simulink model "closed_loop"  (R2019a)
settings: Solver=VariableStepAuto  StartTime=0.0  StopTime=10.0  RelTol=1e-3
values from neighbouring files (symbols this model uses):
  Kp_id = 10    [nomalization.m]
  r = 60    [nomalization.m]
  r_cyc = 4000*ts    (= 200)    [nomalization.m]
libraries: arduinolib x4
settings Model: Creator=xde12  LastModifiedBy=xde12

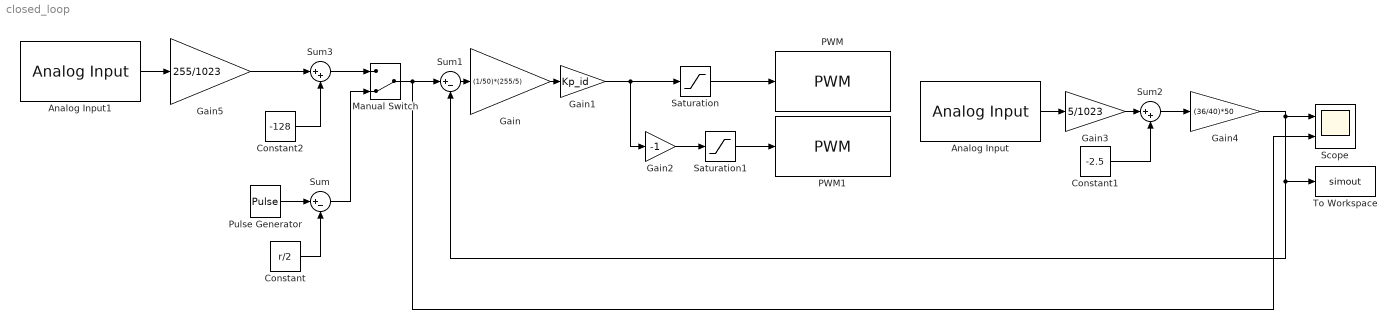
== system closed_loop ==
  Analog Input : arduinolib/Analog Input  pinNumber=0  ReadResultsOnly=off  ConversionTriggerSource=Software  ExternalTriggerType=uint32(0)  OutputDataType=uint16  EnableConversionCompleteNotify=off  EnableOuputStatus=off  SampleTime=0.01  blockPlatform=arduino
  Analog Input1 : arduinolib/Analog Input  pinNumber=0  ReadResultsOnly=off  ConversionTriggerSource=Software  ExternalTriggerType=uint32(0)  OutputDataType=uint16  EnableConversionCompleteNotify=off  EnableOuputStatus=off  SampleTime=0.01  blockPlatform=arduino
  Constant : Constant  Value=r/2  SampleTime=0.01
  Constant1 : Constant  Value=-2.5
  Constant2 : Constant  Value=-128  SampleTime=0.01
  Gain : Gain  Gain=(1/50)*(255/5)
  Gain1 : Gain  Gain=Kp_id
  Gain2 : Gain  Gain=-1
  Gain3 : Gain  Gain=5/1023
  Gain4 : Gain  Gain=(36/40)*50
  Gain5 : Gain  Gain=255/1023
  Manual Switch : ManualSwitch  CurrentSetting=0
  PWM : arduinolib/PWM  pinNumber=3  EnableInputFrequency=off  InitialFrequency=2000  InitialDutyCycle=0  NotificationType=None  blockPlatform=arduino
  PWM1 : arduinolib/PWM  pinNumber=5  EnableInputFrequency=off  InitialFrequency=2000  InitialDutyCycle=0  NotificationType=None  blockPlatform=arduino
  Pulse Generator : DiscretePulseGenerator  PulseType=Time based  Amplitude=r  Period=r_cyc  PulseWidth=r_cyc/2  SampleTime=0.01
  Saturation : Saturate  UpperLimit=255  LowerLimit=0
  Saturation1 : Saturate  UpperLimit=255  LowerLimit=0
  Scope : Scope  NumInputPorts=2
  Sum : Sum  Inputs=|+-
  Sum1 : Sum  Inputs=|+-
  Sum2 : Sum  Inputs=|++
  Sum3 : Sum  Inputs=|++
  To Workspace : ToWorkspace  VariableName=simout  SampleTime=-1
      settings: Save2DSignal=2-D array (concatenate along first dimension)
  wires:
  Pulse Generator/1 -> Sum/1
  Gain/1 -> Gain1/1
  Constant1/1 -> Sum2/2
  Gain2/1 -> Saturation1/1
  Saturation/1 -> PWM/1
  Gain1/1 -> Gain2/1, Saturation/1
  Saturation1/1 -> PWM1/1
  Sum2/1 -> Gain4/1
  Constant/1 -> Sum/2
  Sum1/1 -> Gain/1
  Gain4/1 -> Sum1/2, To Workspace/1, Scope/1
  Analog Input/1 -> Gain3/1
  Gain3/1 -> Sum2/1
  Gain5/1 -> Sum3/1
  Constant2/1 -> Sum3/2
  Analog Input1/1 -> Gain5/1
  Sum3/1 -> Manual Switch/1
  Sum/1 -> Manual Switch/2
  Manual Switch/1 -> Scope/2, Sum1/1
